simulink model "Sri_Lanka_S"  (R2024a)
settings: Solver=VariableStepAuto  StartTime=0.0  StopTime=300  RelTol=1e-3
values from neighbouring files (symbols this model uses):
  D_T = 1500e6/S_base_sys    (= 1.5)    [FUtureGridSL.m]    (also in Sri_Lanka.m; Sri_Lanka_FINAL.m)
  f_base = 50    [FUtureGridSL.m]    (also in Sri_Lanka.m; Sri_Lanka_FINAL.m)
  H_eq = sum(Plant_H .* Plant_S_nom .* Plant_Status) / S_base_sys    [FUtureGridSL.m]    (also in Sri_Lanka.m = sum(Plant_H .* Plant_S_nom) / S_base_sys; Sri_Lanka_FINAL.m = sum(Plant_H .* Plant_S_nom) / S_base_sys)
  LAK_R = 0.04    [FUtureGridSL.m]    (also in Sri_Lanka.m; Sri_Lanka_FINAL.m)
  LAK_S_nom = 300e6    (= 300000000)    [FUtureGridSL.m]    (also in Sri_Lanka.m; Sri_Lanka_FINAL.m)
  RHT_F_HP = 0.3    [FUtureGridSL.m]    (also in Sri_Lanka.m; Sri_Lanka_FINAL.m)
  RHT_T_CH = 0.3    [FUtureGridSL.m]    (also in Sri_Lanka.m; Sri_Lanka_FINAL.m)
  RHT_T_RH = 7.0    (= 7)    [FUtureGridSL.m]    (also in Sri_Lanka.m; Sri_Lanka_FINAL.m)
  rocof_meas_window = 0.18    [FUtureGridSL.m]    (also in Sri_Lanka.m; Sri_Lanka_FINAL.m)
  S_base_sys = 1000e6    (= 1000000000)    [FUtureGridSL.m]    (also in Sri_Lanka.m; Sri_Lanka_FINAL.m)
  SAM_R_P = 0.05    [FUtureGridSL.m]    (also in Sri_Lanka.m; Sri_Lanka_FINAL.m)
  SAM_R_T = 0.38    [FUtureGridSL.m]    (also in Sri_Lanka.m; Sri_Lanka_FINAL.m)
  SAM_T_R = 5.0    (= 5)    [FUtureGridSL.m]    (also in Sri_Lanka.m; Sri_Lanka_FINAL.m)
  SAM_T_W = 1.5    [FUtureGridSL.m]    (also in Sri_Lanka.m; Sri_Lanka_FINAL.m)
  SAM_Unit_S_nom = 60e6    (= 60000000)    [FUtureGridSL.m]    (also in Sri_Lanka.m; Sri_Lanka_FINAL.m)
  t_dist = 200    [FUtureGridSL.m]    (also in Sri_Lanka.m; Sri_Lanka_FINAL.m)
  T_G = 0.2    [FUtureGridSL.m]    (also in Sri_Lanka.m; Sri_Lanka_FINAL.m)
settings Model: Creator=munas  LastModifiedBy=munas

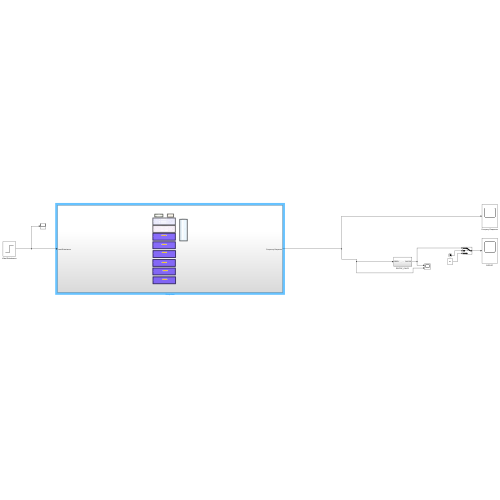
[thumbnail: Simulink's stored preview of the top-level diagram]
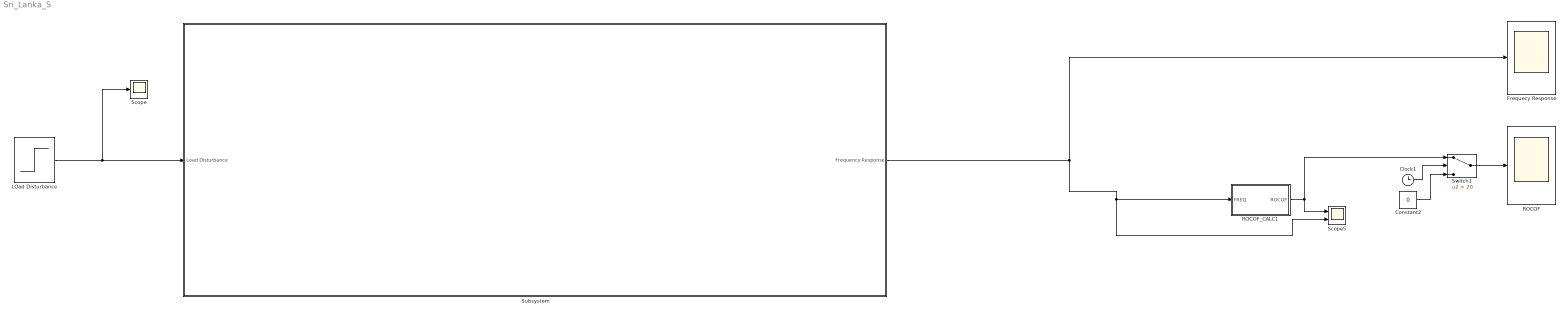
== system Sri_Lanka_S ==
  Clock1 : Clock
  Constant2 : Constant  Value=0
  Frequecy Response : Scope
  LOad Disturbance : Step  Time=t_dist  After=0.05  SampleTime=0
  ROCOF : Scope
  ROCOF_CALC1 : Subsystem
  Scope : Scope
  Scope5 : Scope  NumInputPorts=2
  Subsystem : Subsystem
  Switch1 : Switch  Criteria=u2 > Threshold  Threshold=20  SaturateOnIntegerOverflow=off  InputSameDT=off
  wires:
  LOad Disturbance/1 -> Subsystem/1(Load Disturbance), Scope/1
  Subsystem/1(Frequency Response) -> Scope5/2, ROCOF_CALC1/1(FREQ), Frequecy Response/1
  Constant2/1 -> Switch1/3
  Switch1/1 -> ROCOF/1
  Clock1/1 -> Switch1/2
  ROCOF_CALC1/1(ROCOF) -> Switch1/1, Scope5/1

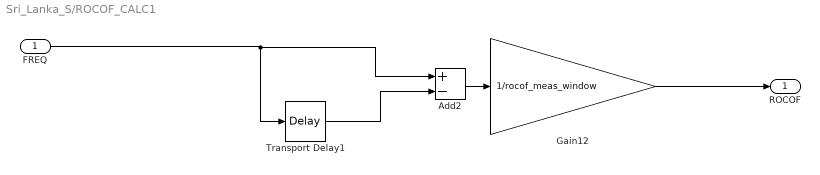
== system Sri_Lanka_S/ROCOF_CALC1 ==
  FREQ : Inport
  Add2 : Sum  Inputs=+-
  Gain12 : Gain  Gain=1/rocof_meas_window
  Transport Delay1 : TransportDelay  DelayTime=rocof_meas_window  InitialOutput=50
  ROCOF : Outport
  wires:
  Transport Delay1/1 -> Add2/2
  Gain12/1 -> ROCOF/1
  Add2/1 -> Gain12/1
  FREQ/1 -> Add2/1, Transport Delay1/1

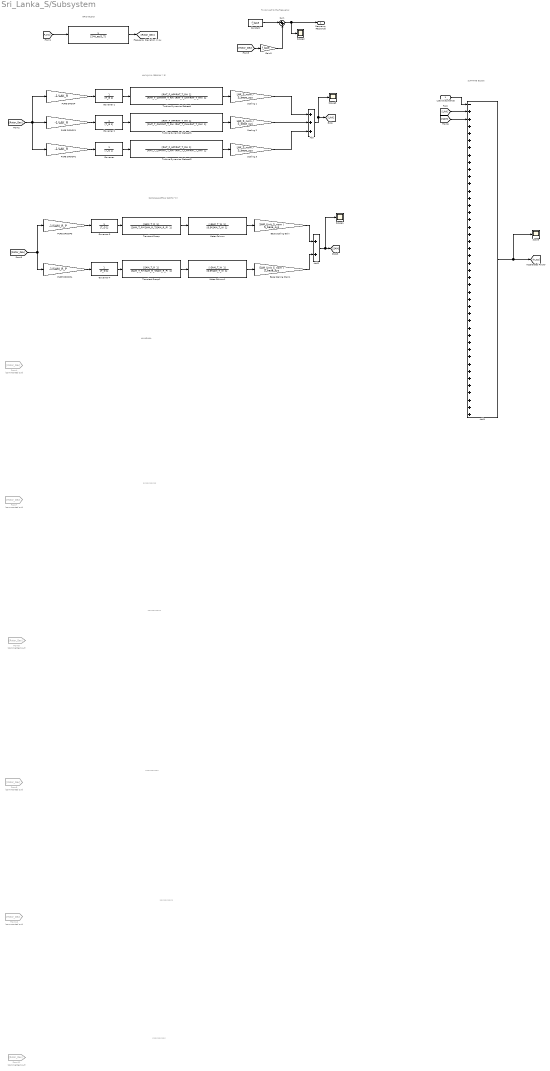
== system Sri_Lanka_S/Subsystem ==
  note: SAMANALAWEWA (60MW *2 )
  note: GRID BLOCK
  note: SUMMING BLOCK
  note: To convert to the frequency
  note: LAKVIJAYA (300MW * 3)
  note: LAXAPANA
  note: xxxxxxxxxx
  note: xxxxxxxxxx
  note: xxxxxxxxxx
  note: xxxxxxxxxx
  note: xxxxxxxxxx
  Load Disturbance : Inport
  " " : TransferFcn  Denominator=[2*H_eq D_T]
  Add : Sum  Inputs=+++
  Add1 : Sum  Inputs=-+++++++++++++++++++++++++++++++++++++++++++
  Add2 : Sum
  Base Scaling Gain : Gain  Gain=SAM_Unit_S_nom / S_base_sys
  Base Scaling Gain1 : Gain  Gain=SAM_Unit_S_nom / S_base_sys
  Constant : Constant  Value=f_base
  From{4,7..11} (6 alike) : From  Commented=on  GotoTag=Rotor_Dev
  Gain3 : Gain  Gain=f_base
  Governer : TransferFcn  Denominator=[T_G 1]
  Governer {1..4} (4 alike) : TransferFcn  Denominator=[T_G 1]
  PURE DROOP : Gain  Gain=-1/LAK_R
  PURE DROOP1 : Gain  Gain=-1/LAK_R
  PURE DROOP2 : Gain  Gain=-1/LAK_R
  PURE DROOP3 : Gain  Gain=-1/SAM_R_P
  PURE DROOP4 : Gain  Gain=-1/SAM_R_P
  Scaling 1 : Gain  Gain=LAK_S_nom / S_base_sys
  Scaling 2 : Gain  Gain=LAK_S_nom / S_base_sys
  Scaling 3 : Gain  Gain=LAK_S_nom / S_base_sys
  Scope{,1..3} (4 alike) : Scope
  Sum : Sum  Inputs=|++
  Transient Droop : TransferFcn  Numerator="[SAM_T_R  1]"  Denominator="[SAM_T_R*(SAM_R_T/SAM_R_P)  1]"
  Transient Droop1 : TransferFcn  Numerator="[SAM_T_R  1]"  Denominator="[SAM_T_R*(SAM_R_T/SAM_R_P)  1]"
  Turbine Dynamics (Reheat) : TransferFcn  Numerator="[RHT_F_HP*RHT_T_RH  1]"  Denominator="[RHT_T_CH*RHT_T_RH  (RHT_T_CH+RHT_T_RH)  1]"
  Turbine Dynamics (Reheat)1 : TransferFcn  Numerator="[RHT_F_HP*RHT_T_RH  1]"  Denominator="[RHT_T_CH*RHT_T_RH  (RHT_T_CH+RHT_T_RH)  1]"
  Turbine Dynamics (Reheat)2 : TransferFcn  Numerator="[RHT_F_HP*RHT_T_RH  1]"  Denominator="[RHT_T_CH*RHT_T_RH  (RHT_T_CH+RHT_T_RH)  1]"
  Water Column : TransferFcn  Numerator="[-SAM_T_W  1]"  Denominator="[0.5*SAM_T_W  1]"
  Water Column1 : TransferFcn  Numerator="[-SAM_T_W  1]"  Denominator="[0.5*SAM_T_W  1]"
  Frequency Response : Outport
  wires:
  Governer 1/1 -> Turbine Dynamics (Reheat)/1
  Turbine Dynamics (Reheat)/1 -> Scaling 1/1
  PURE DROOP/1 -> Governer 1/1
  Sum/1 -> Scope2/1, Frequency Response/1
  Constant/1 -> Sum/1
  Scaling 1/1 -> Add/1
  PURE DROOP1/1 -> Governer 2/1
  Governer 2/1 -> Turbine Dynamics (Reheat)1/1
  Turbine Dynamics (Reheat)1/1 -> Scaling 2/1
  Scaling 2/1 -> Add/2
  Governer/1 -> Turbine Dynamics (Reheat)2/1
  PURE DROOP2/1 -> Governer/1
  Turbine Dynamics (Reheat)2/1 -> Scaling 3/1
  Scaling 3/1 -> Add/3
  Add/1 -> Scope3/1, [LAK]
  [P_acc] -> " "/1
  " "/1 -> [Rotor_Dev]
  [Rotor_Dev] -> PURE DROOP2/1, PURE DROOP/1, PURE DROOP1/1
  [Rotor_Dev] -> Gain3/1
  [LAK] -> Add1/2
  Add1/1 -> Scope/1, [P_acc]
  Load Disturbance/1 -> Add1/1
  [Rotor_Dev] -> PURE DROOP4/1, PURE DROOP3/1
  PURE DROOP3/1 -> Governer 3/1
  Base Scaling Gain/1 -> Add2/1
  Governer 3/1 -> Transient Droop/1
  Add2/1 -> Scope1/1, [SAM]
  Transient Droop/1 -> Water Column/1
  Water Column/1 -> Base Scaling Gain/1
  Water Column1/1 -> Base Scaling Gain1/1
  Transient Droop1/1 -> Water Column1/1
  Governer 4/1 -> Transient Droop1/1
  PURE DROOP4/1 -> Governer 4/1
  Base Scaling Gain1/1 -> Add2/2
  [SAM] -> Add1/3
  Gain3/1 -> Sum/2
